simulink model "sparse_bayes_filter2"  (R2021b)
settings: Solver=FixedStepDiscrete  StartTime=0.0  StopTime=100.0  FixedStep=0.01  RelTol=1e-3
libraries: wnnlib x28
settings Model: Creator=20214358  LastModifiedBy=20214358
settings HardwareCC: ProdLongLongMode=on  TargetBitPerPointer=64  TargetBitPerSizeT=64  TargetBitPerPtrDiffT=64  TargetLargestAtomicFloat=Float  TargetIntDivRoundTo=Zero  TargetEndianess=LittleEndian  TargetWordSize=64  TargetHWDeviceType=Intel->x86-64 (Windows64)

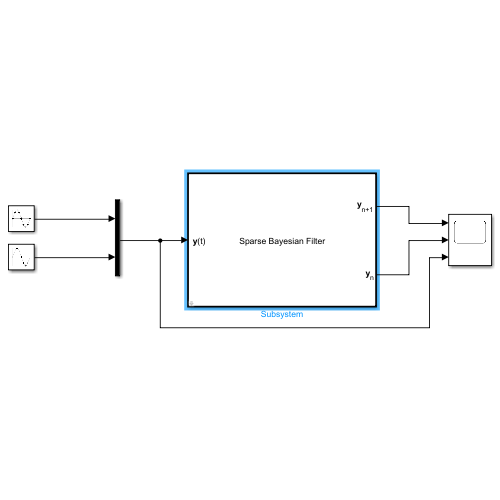
[thumbnail: Simulink's stored preview of the top-level diagram]
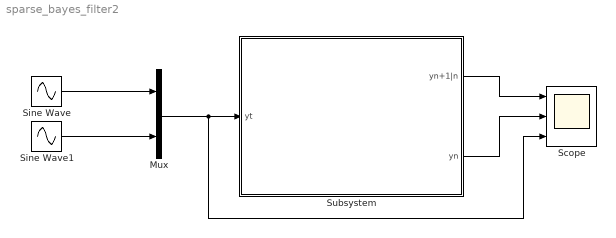
== system sparse_bayes_filter2 ==
  Mux : Mux  Inputs=2
  Scope : Scope  NumInputPorts=3
  Sine Wave : Sin  SineType=Sample based  Amplitude=5  Samples=1100  SampleTime=0.01
  Sine Wave1 : Sin  SineType=Sample based  Amplitude=5  Phase=1  Samples=1100  SampleTime=0.01  Offset=275
  Subsystem : Subsystem  TreatAsAtomicUnit=on  mask{filter_match_tolerance=1, filter_number_of_random_flips=96, observation_dense_vector_length=2, observation_sparse_vector_length=2048, observation_memory_size=[511 512], observation_hamming_distance=[2 64], observation_vgram_array_length=16384, observation_number_of_samples=96, dynamics_memory_size=[511 512], dynamics_hamming_distance=[2 64], dynamics_vgram_array_length=4096, dynamics_number_of_samples=96, codec_number_of_sparse_vectors=16384, codec_learning_rate=0.00000000000000000000001, codec_min_bounds=[-10 -10], codec_max_bounds=[10 10], codec_sparse_vectors_file='C:\Users\20214358\MATLAB\Projects\wnnlib\wnndata\16k_sparse_vectors_seed_0.npz'}
      mask prompts: filter_match_tolerance "Match tolerance"; filter_number_of_random_flips "Number of random flips"; observation_dense_vector_length "Dense vector length"; observation_sparse_vector_length "Sparse vector length"; observation_memory_size "Memory size"; observation_hamming_distance "Hamming distance"; observation_vgram_array_length "VGRAM array length"; observation_number_of_samples "Number of samples"; dynamics_memory_size "Memory size"; dynamics_hamming_distance "Hamming distance"; dynamics_vgram_array_length "VGRAM array length"; dynamics_number_of_samples "Number of samples"; codec_number_of_sparse_vectors "Number of sparse vectors"; codec_learning_rate "Learning rate"; codec_min_bounds "Minimum bounds"; codec_max_bounds "Maximum bounds"; codec_sparse_vectors_file "Sparse vectors file"
      mask init:
      | codec_max_kdtree_depth = ceil(log2(codec_number_of_sparse_vectors));
      | codec_min_splitting_volume = prod(codec_max_bounds - codec_min_bounds)/codec_number_of_sparse_vectors;
      | codec_sparse_vectors_file = char(codec_sparse_vectors_file);
      mask DialogControl FilterParams Prompt: Filter
      mask DialogControl ObservationModelParams Prompt: Observation model
      mask DialogControl DynamicModelParams Prompt: Dynamic model
      mask DialogControl CodecParams Prompt: Codec
      mask Display:
      | disp('Sparse Bayesian Filter','interpreter','tex');
      | port_label('input', 1,'{\bf y}(t)','interpreter','tex');
      | port_label('output', 1,'{\bf y}_{n+1}','interpreter','tex');
      | port_label('output', 2,'{\bf y}_{n}','interpreter','tex');
  wires:
  Subsystem/1(yn+1|n) -> Scope/1
  Mux/1 -> Scope/3, Subsystem/1(yt)
  Sine Wave/1 -> Mux/1
  Sine Wave1/1 -> Mux/2
  Subsystem/2(yn) -> Scope/2

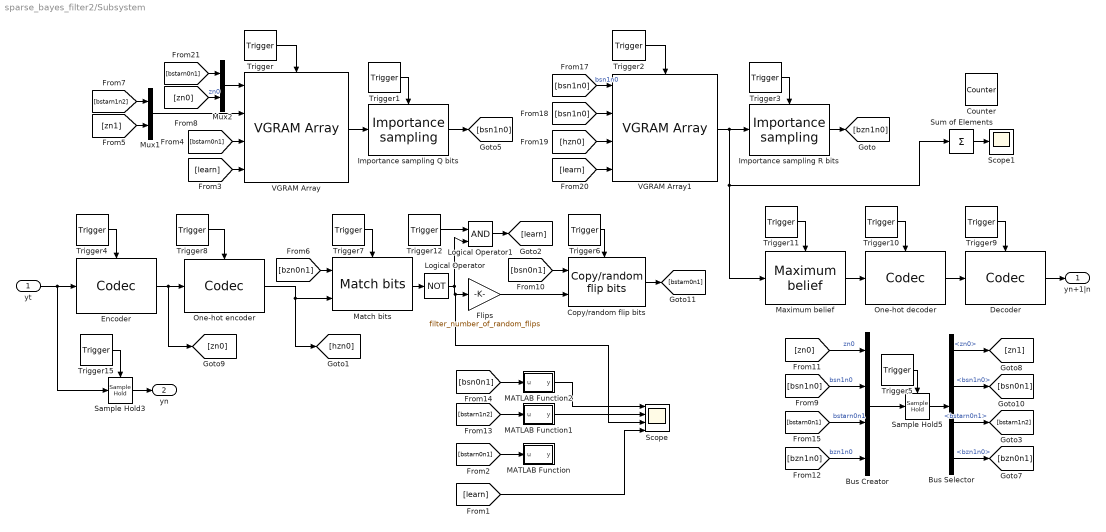
== system sparse_bayes_filter2/Subsystem ==
  yt : Inport
  Bus Creator : BusCreator  Inputs=4
  Bus Selector : BusSelector  OutputSignals=zn0,bsn1n0,bstarn0n1,bzn1n0
  Copy/random flip bits : wnnlib/Utilities/Copy//random flip bits
      settings: SourceProductName=Weightless Neural Networks Toolbox
  Counter : wnnlib/Sources/Counter  number_of_steps=10  sample_time=-1
      settings: SourceProductName=Weightless Neural Networks Toolbox
  Decoder : wnnlib/Utilities/Codec  codec_id=0  dense_vector_length=observation_dense_vector_length  sparse_vector_length=observation_sparse_vector_length  max_depth=codec_max_kdtree_depth  learning_rate=codec_learning_rate  min_splitting_volume=codec_min_splitting_volume  min_bounds=codec_min_bounds  max_bounds=codec_max_bounds  sparse_vectors_file=codec_sparse_vectors_file  debug_flag=off  codec_type=Decoder  number_of_sparse_vectors=65536
      settings: SourceProductName=Weightless Neural Networks Toolbox
  Encoder : wnnlib/Utilities/Codec  codec_id=0  dense_vector_length=observation_dense_vector_length  sparse_vector_length=observation_sparse_vector_length  max_depth=codec_max_kdtree_depth  learning_rate=codec_learning_rate  min_splitting_volume=codec_min_splitting_volume  min_bounds=codec_min_bounds  max_bounds=codec_max_bounds  sparse_vectors_file=codec_sparse_vectors_file  debug_flag=off  codec_type=Encoder  number_of_sparse_vectors=65536
      settings: SourceProductName=Weightless Neural Networks Toolbox
  Flips : Gain  Gain=filter_number_of_random_flips  OutDataTypeStr=uint8
  Importance sampling Q bits : wnnlib/Utilities/Importance sampling  nSamples=dynamics_number_of_samples
      settings: SourceProductName=Weightless Neural Networks Toolbox
  Importance sampling R bits : wnnlib/Utilities/Importance sampling  nSamples=observation_number_of_samples
      settings: SourceProductName=Weightless Neural Networks Toolbox
  Logical Operator : Logic  Operator=NOT  IconShape=distinctive  AllPortsSameDT=off  OutDataTypeStr=boolean
  Logical Operator1 : Logic  IconShape=distinctive  AllPortsSameDT=off  OutDataTypeStr=boolean
  MATLAB Function : MATLAB Function  TreatAsAtomicUnit=on
  MATLAB Function1 : MATLAB Function  TreatAsAtomicUnit=on
  MATLAB Function2 : MATLAB Function  TreatAsAtomicUnit=on
  Match bits : wnnlib/Utilities/Match bits  nMatchTolerance=filter_match_tolerance
      settings: SourceProductName=Weightless Neural Networks Toolbox
  Maximum belief : wnnlib/Utilities/Maximum belief  SystemSampleTime=-1  VariantActivationTime=update diagram  Latency=0  AutoFrameSizeCalculation=off
      settings: SourceProductName=Weightless Neural Networks Toolbox
  Mux1 : Mux  Inputs=2
  Mux2 : Mux  Inputs=2
  One-hot decoder : wnnlib/Utilities/Codec  codec_id=0  dense_vector_length=observation_dense_vector_length  sparse_vector_length=observation_sparse_vector_length  max_depth=codec_max_kdtree_depth  learning_rate=codec_learning_rate  min_splitting_volume=codec_min_splitting_volume  min_bounds=codec_min_bounds  max_bounds=codec_max_bounds  sparse_vectors_file=codec_sparse_vectors_file  debug_flag=off  codec_type=OneHotDecoder  number_of_sparse_vectors=codec_number_of_sparse_vectors
      settings: SourceProductName=Weightless Neural Networks Toolbox
  One-hot encoder : wnnlib/Utilities/Codec  codec_id=0  dense_vector_length=observation_dense_vector_length  sparse_vector_length=observation_sparse_vector_length  max_depth=codec_max_kdtree_depth  learning_rate=codec_learning_rate  min_splitting_volume=codec_min_splitting_volume  min_bounds=codec_min_bounds  max_bounds=codec_max_bounds  sparse_vectors_file=codec_sparse_vectors_file  debug_flag=off  codec_type=OneHotEncoder  number_of_sparse_vectors=codec_number_of_sparse_vectors
      settings: SourceProductName=Weightless Neural Networks Toolbox
  Sample Hold3 : wnnlib/Utilities/Sample Hold  sample_time=-1
      settings: SourceProductName=Weightless Neural Networks Toolbox
  Sample Hold5 : wnnlib/Utilities/Sample Hold  sample_time=-1
      settings: SourceProductName=Weightless Neural Networks Toolbox
  Scope : Scope  NumInputPorts=4
  Scope1 : Scope
  Sum of Elements : Sum  Inputs=+
  Trigger : wnnlib/Sources/Trigger  selected_steps=[4 5]
      settings: SourceProductName=Weightless Neural Networks Toolbox
  Trigger1 : wnnlib/Sources/Trigger  selected_steps=[5 6]
      settings: SourceProductName=Weightless Neural Networks Toolbox
  Trigger10 : wnnlib/Sources/Trigger  selected_steps=[8 9]
      settings: SourceProductName=Weightless Neural Networks Toolbox
  Trigger11 : wnnlib/Sources/Trigger  selected_steps=[7 8]
      settings: SourceProductName=Weightless Neural Networks Toolbox
  Trigger12 : wnnlib/Sources/Trigger  selected_steps=[4 6]
      settings: SourceProductName=Weightless Neural Networks Toolbox
  Trigger15 : wnnlib/Sources/Trigger  selected_steps=0
      settings: SourceProductName=Weightless Neural Networks Toolbox
  Trigger2 : wnnlib/Sources/Trigger  selected_steps=[6 7]
      settings: SourceProductName=Weightless Neural Networks Toolbox
  Trigger3 : wnnlib/Sources/Trigger  selected_steps=8
      settings: SourceProductName=Weightless Neural Networks Toolbox
  Trigger4 : wnnlib/Sources/Trigger  selected_steps=0
      settings: SourceProductName=Weightless Neural Networks Toolbox
  Trigger5 : wnnlib/Sources/Trigger  selected_steps=10
      settings: SourceProductName=Weightless Neural Networks Toolbox
  Trigger6 : wnnlib/Sources/Trigger  selected_steps=3
      settings: SourceProductName=Weightless Neural Networks Toolbox
  Trigger7 : wnnlib/Sources/Trigger  selected_steps=2
      settings: SourceProductName=Weightless Neural Networks Toolbox
  Trigger8 : wnnlib/Sources/Trigger  selected_steps=1
      settings: SourceProductName=Weightless Neural Networks Toolbox
  Trigger9 : wnnlib/Sources/Trigger  selected_steps=[9 10]
      settings: SourceProductName=Weightless Neural Networks Toolbox
  VGRAM Array : wnnlib/Models/VGRAM Array  array_id=0  min_mem_size=dynamics_memory_size(1)  max_mem_size=dynamics_memory_size(2)  min_dist=dynamics_hamming_distance(1)  max_dist=dynamics_hamming_distance(2)  pattern_length=dynamics_vgram_array_length+observation_sparse_vector_length  output_dims=[dynamics_vgram_array_length 1]  debug_flag=off
      settings: SourceProductName=Weightless Neural Networks Toolbox
  VGRAM Array1 : wnnlib/Models/VGRAM Array  array_id=1  min_mem_size=observation_memory_size(1)  max_mem_size=observation_memory_size(2)  min_dist=observation_hamming_distance(1)  max_dist=observation_hamming_distance(2)  pattern_length=dynamics_vgram_array_length  output_dims=[observation_vgram_array_length 1]  debug_flag=off
      settings: SourceProductName=Weightless Neural Networks Toolbox
  yn+1|n : Outport
  yn : Outport  Port=2
  wires:
  Trigger1/1 -> Importance sampling Q bits/Trigger
  Trigger2/1 -> VGRAM Array1/Trigger
  VGRAM Array/1 -> Importance sampling Q bits/1
  Trigger4/1 -> Encoder/Trigger
  Trigger7/1 -> Match bits/Trigger
  Trigger6/1 -> Copy/random flip bits/Trigger
  Match bits/1 -> Logical Operator/1
  Trigger/1 -> VGRAM Array/Trigger
  Trigger3/1 -> Importance sampling R bits/Trigger
  [bzn0n1] -> Match bits/1
  Logical Operator/1 -> Logical Operator1/2, Scope/3, Flips/1
  Importance sampling R bits/1 -> [bzn1n0]
  Trigger8/1 -> One-hot encoder/Trigger
  [bsn0n1] -> Copy/random flip bits/1
  Copy/random flip bits/1 -> [bstarn0n1]
  [bsn1n0] -> VGRAM Array1/2
  Decoder/1 -> yn+1|n/1
  Trigger9/1 -> Decoder/Trigger
  One-hot decoder/1 -> Decoder/1
  Trigger10/1 -> One-hot decoder/Trigger
  Trigger11/1 -> Maximum belief/Trigger
  Trigger12/1 -> Logical Operator1/1
  Logical Operator1/1 -> [learn]
  [learn] -> VGRAM Array1/4
  VGRAM Array1/1 -> Maximum belief/1, Sum of Elements/1, Importance sampling R bits/1
  [learn] -> VGRAM Array/4
  yt/1 -> Encoder/1, Sample Hold3/1
  Encoder/1 -> [zn0], One-hot encoder/1
  Importance sampling Q bits/1 -> [bsn1n0]
  [bstarn0n1] -> Mux2/1
  Trigger15/1 -> Sample Hold3/Trigger
  Sample Hold3/1 -> yn/1
  Mux1/1 -> VGRAM Array/2
  [bstarn1n2] -> Mux1/1
  [zn1] -> Mux1/2
  Trigger5/1 -> Sample Hold5/Trigger
  Bus Creator/1 -> Sample Hold5/1
  Sample Hold5/1 -> Bus Selector/1
  [zn0] -> Bus Creator/1  "zn0"
  Bus Selector/1 -> [zn1]  "<zn0>"
  Bus Selector/2 -> [bsn0n1]  "<bsn1n0>"
  Bus Selector/3 -> [bstarn1n2]  "<bstarn0n1>"
  Bus Selector/4 -> [bzn0n1]  "<bzn1n0>"
  [bsn1n0] -> Bus Creator/2  "bsn1n0"
  [bstarn0n1] -> Bus Creator/3  "bstarn0n1"
  [bzn1n0] -> Bus Creator/4  "bzn1n0"
  Maximum belief/1 -> One-hot decoder/1
  Mux2/1 -> VGRAM Array/1
  [zn0] -> Mux2/2  "zn0"
  [bsn1n0] -> VGRAM Array1/1  "bsn1n0"
  One-hot encoder/1 -> Match bits/2, [hzn0]
  [learn] -> Scope/4
  [bstarn0n1] -> MATLAB Function/1(u)
  [bstarn1n2] -> MATLAB Function1/1(u)
  [bsn0n1] -> MATLAB Function2/1(u)
  Flips/1 -> Copy/random flip bits/2
  MATLAB Function2/1(y) -> Scope/1
  MATLAB Function1/1(y) -> Scope/2
  [bstarn0n1] -> VGRAM Array/3
  [hzn0] -> VGRAM Array1/3
  Sum of Elements/1 -> Scope1/1

== matlab function sparse_bayes_filter2/Subsystem/MATLAB Function ==
  data: u input; y output
function y = fcn(u)
y=0;
for i=1:length(u)
    if u(i) ~= 0
        y = y+i;
    end
end

== matlab function sparse_bayes_filter2/Subsystem/MATLAB Function2 ==
  data: u input; y output
function y = fcn(u)
y=0;
for i=1:length(u)
    if u(i) ~= 0
        y = y+i;
    end
end

== matlab function sparse_bayes_filter2/Subsystem/MATLAB Function1 ==
  data: u input; y output
function y = fcn(u)
y=0;
for i=1:length(u)
    if u(i) ~= 0
        y = y+i;
    end
end
